simulink model "LQRD"  (R2015a)
settings: Solver=ode3  StartTime=0.0  StopTime=10.0  FixedStep=0.02  RelTol=1e-3
values from neighbouring files (symbols this model uses):
  Ad = expm(A*T)    [CubliFunction.m]
  Bd = inv(A)*(Ad-eye(3))*B    [CubliFunction.m]
  C = eye(3)    [CubliFunction.m]
  Kd1 = Kd(1,1)    [CubliFunction.m]
  Kd2 = Kd(1,2)    [CubliFunction.m]
  Kd3 = Kd(1,3)    [CubliFunction.m]
settings Model: Creator=Remy  LastModifiedBy=Remy

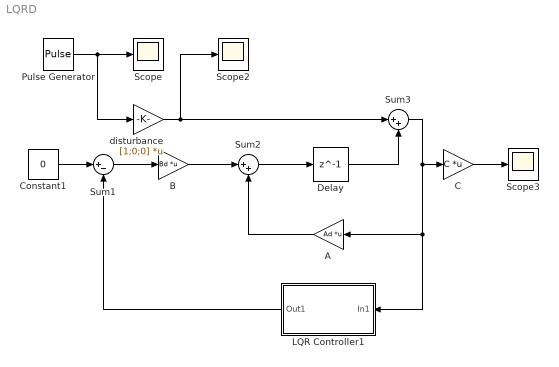
== system LQRD ==
  A : Gain  Gain=Ad  Multiplication=Matrix(K*u) (u vector)
  B : Gain  Gain=Bd  Multiplication=Matrix(K*u)
  C : Gain  Gain=C  Multiplication=Matrix(K*u)
  Constant1 : Constant  Value=0
  Delay : Delay  DelayLength=1
  LQR Controller1 : Subsystem  mask(LQR Controller){K1=Kd1, K2=Kd2, K3=Kd3}
  Pulse Generator : DiscretePulseGenerator  PulseType=Time based  Amplitude=0.1  Period=10  PulseWidth=0.2  PhaseDelay=1
  Scope : Scope
  Scope2 : Scope
      settings: ShowLegends=on  SaveName=ScopeData2
  Scope3 : Scope
      settings: ShowLegends=on  SaveName=ScopeData3
  Sum1 : Sum  Inputs=|+-
  Sum2 : Sum  Inputs=|++
  Sum3 : Sum  Inputs=|++
  disturbance : Gain  Gain=[1;0;0]  Multiplication=Matrix(K*u)
  wires:
  Constant1/1 -> Sum1/1
  Sum1/1 -> B/1
  Sum2/1 -> Delay/1
  Delay/1 -> Sum3/2
  B/1 -> Sum2/1
  Sum3/1 -> LQR Controller1/1(In1), A/1, C/1
  C/1 -> Scope3/1
  A/1 -> Sum2/2
  LQR Controller1/1(Out1) -> Sum1/2
  Pulse Generator/1 -> Scope/1, disturbance/1
  disturbance/1 -> Sum3/1, Scope2/1

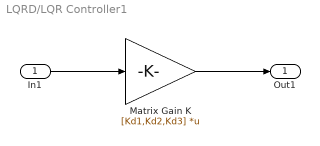
== system LQRD/LQR Controller1 ==
  In1 : Inport
  Matrix Gain K : Gain  Gain=[Kd1,Kd2,Kd3]  Multiplication=Matrix(K*u)
  Out1 : Outport
  wires:
  In1/1 -> Matrix Gain K/1
  Matrix Gain K/1 -> Out1/1
